simulink model "cartpole_balance"  (R2023b)
settings: Solver=FixedStepAuto  StartTime=0.0  StopTime=20  FixedStep=0.01  RelTol=1e-3
settings Model: Creator=gomes  LastModifiedBy=gomes
settings SolverCC: AlgebraicLoopSolver=TrustRegion
settings DebuggingCC: UnconnectedInputMsg=warning  UnconnectedOutputMsg=warning  UnconnectedLineMsg=warning
settings ModelReferenceCC: EnableRefExpFcnMdlSchedulingChecks=on
settings RTWCC: DLArmComputeVersion=19.05

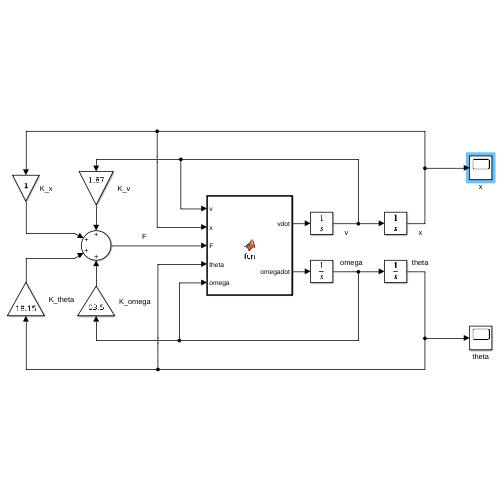
[thumbnail: Simulink's stored preview of the top-level diagram]
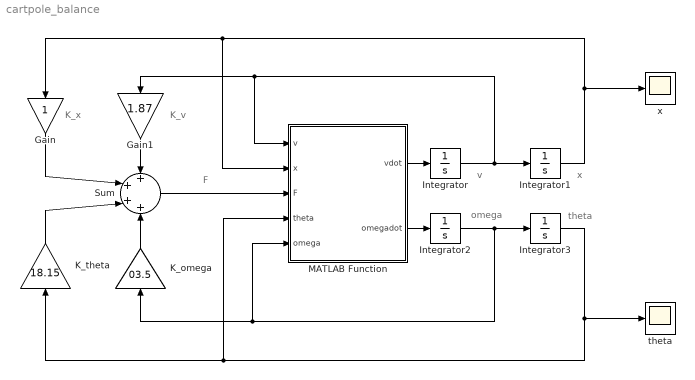
== system cartpole_balance ==
  note: x
  note: v
  note: omega
  note: theta
  note: K_v
  note: K_x
  note: F
  Gain : Gain
  Gain1 : Gain  Gain=1.87
  Integrator : Integrator
  Integrator1 : Integrator
  Integrator2 : Integrator
  Integrator3 : Integrator  InitialCondition=0.1
  K_omega : Gain  Gain=03.5
  K_theta : Gain  Gain=18.15
  MATLAB Function : MATLAB Function  TreatAsAtomicUnit=on
  Sum : Sum  Inputs=++++
  theta : Scope
  x : Scope
  wires:
  Integrator2/1 -> MATLAB Function/5(omega), K_omega/1, Integrator3/1
  Integrator/1 -> Gain1/1, MATLAB Function/1(v), Integrator1/1
  Integrator1/1 -> MATLAB Function/2(x), Gain/1, x/1
  Integrator3/1 -> MATLAB Function/4(theta), K_theta/1, theta/1
  MATLAB Function/1(vdot) -> Integrator/1
  MATLAB Function/2(omegadot) -> Integrator2/1
  Sum/1 -> MATLAB Function/3(F)
  Gain/1 -> Sum/2
  K_omega/1 -> Sum/4
  Gain1/1 -> Sum/1
  K_theta/1 -> Sum/3

== matlab function cartpole_balance/MATLAB Function ==
  data: v input; x input; vdot output; omegadot output; F input; theta input; omega input
function [vdot,omegadot] = fcn(v,x,F,theta,omega)

m = 0.2;
M = 0.4;
l = 0.3;
g = 9.8;

btheta = 0.2;
bx = 0.2;

ct = cos(theta);
st = sin(theta);

A = [ct , 4*l/3 ; M+m  ,m*l*ct];
b = [st*g-btheta*omega ; m*l*st*omega^2+F-bx*v];

sol = A\b;

vdot     = sol(1);
omegadot = sol(2);
